simulink model "lab3"  (R2021b)
settings: Solver=ode45  StartTime=0.0  StopTime=500  RelTol=1e-3  EnableMultiTasking=on
settings Model: Creator=user  LastModifiedBy=Lapte
settings SolverCC: AlgebraicLoopSolver=TrustRegion
settings DataIOCC: LimitDataPoints=on  SaveFormat=Array  ReturnWorkspaceOutputs=off
settings OptimizationCC: LifeSpan=inf
settings DebuggingCC: SolverPrmCheckMsg=warning  SFUnexpectedBacktrackingDiag=warning  SFNoUnconditionalDefaultTransitionDiag=warning  SFExecutionAtInitializationDiag=none  SFMachineParentedDataDiag=warning  ArithmeticOperatorsInVariantConditions=warning
settings HardwareCC: ProdBitPerPointer=32  ProdBitPerSizeT=32  ProdBitPerPtrDiffT=32  ProdLargestAtomicFloat=None  ProdIntDivRoundTo=Undefined  ProdEndianess=Unspecified  ProdWordSize=32  ProdHWDeviceType=32-bit Generic
settings ModelReferenceCC: PropagateSignalLabelsOutOfModel=off
settings SFSimCC: SimUseLocalCustomCode=off  CustomCodeUndefinedFunction=UseInterfaceOnly
settings RTWCC: RTWUseLocalCustomCode=off
settings CodeAppCC: StateflowObjectComments=on
settings GRTTargetCC: TargetLangStandard=C89/C90 (ANSI)
settings ConfigComp: CovMetricSettings=dw  CovSaveCumulativeToWorkspaceVar=on  CovSaveSingleToWorkspaceVar=on  CovExternalEMLEnable=off  CovSFcnEnable=off

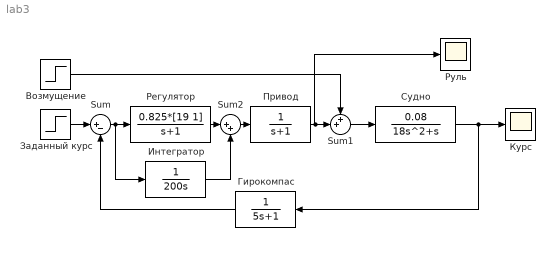
== system lab3 ==
  Sum : Sum  Inputs=|+-
  Sum1 : Sum  Inputs=++|
  Sum2 : Sum  Inputs=|++
  Возмущение : Step  Time=0  After=2  SampleTime=0
  Гирокомпас : TransferFcn  Denominator=[5 1]
  Заданный курс : Step  Time=0  After=10  SampleTime=0
  Интегратор : TransferFcn  Denominator=[200 0]
  Курс : Scope
  Привод : TransferFcn  Denominator=[1 1]
  Регулятор : TransferFcn  Numerator=0.825*[19 1]  Denominator=[1 1]
  Руль : Scope
  Судно : TransferFcn  Numerator=[0.08]  Denominator=[18 1 0]
  wires:
  Заданный курс/1 -> Sum/1
  Sum/1 -> Интегратор/1, Регулятор/1
  Судно/1 -> Курс/1, Гирокомпас/1
  Гирокомпас/1 -> Sum/2
  Возмущение/1 -> Sum1/1
  Привод/1 -> Руль/1, Sum1/2
  Sum1/1 -> Судно/1
  Регулятор/1 -> Sum2/1
  Sum2/1 -> Привод/1
  Интегратор/1 -> Sum2/2
